simulink model "Wanderwellen_Leitungsmodell"  (R2022a)
settings: Solver=VariableStepAuto  StartTime=0.0  StopTime=0.05  RelTol=1e-3
model workspace (MAT data in the model file):
  C_impedanz = 1
  C_quelle = 1
  Delta_C = 2e-09
  Delta_G = 5000000
  Delta_L = 0.000228
  Delta_R = 0.048
  L_impedanz = 1
  L_quelle = 1
  R_impedanz = 0
  R_quelle = 0
  U = 20000
  U_type = 1
  Z_abschluss_type = 1
  Z_quelle_type = 1
  f = 50
  laenge = 0.2
  n_seg = 1
libraries: fl_lib x617, nesl_utility x207, ee_lib x3
(part 2 of 6)

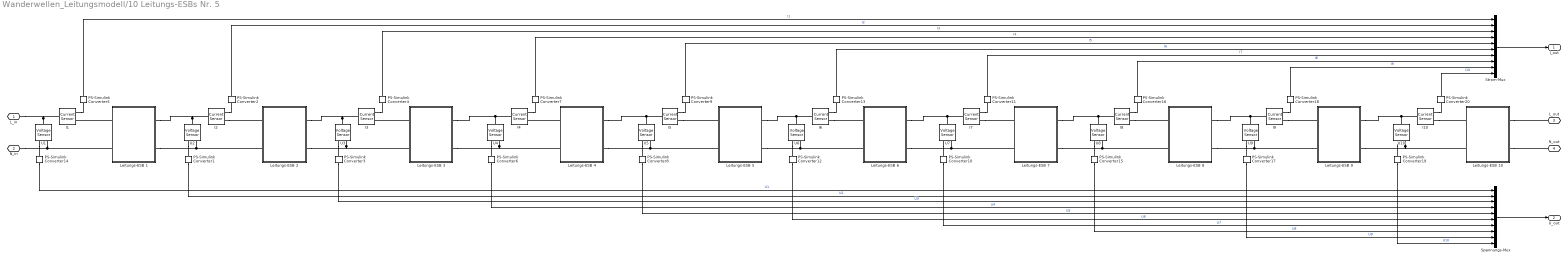
== system Wanderwellen_Leitungsmodell/10 Leitungs-ESBs Nr. 5 ==
  I{1..10} (10 alike) : fl_lib/Electrical/Electrical Sensors/Current Sensor
      settings: SourceProductBaseCode=PW,SS,VE
  Leitungs-ESB 1 : Subsystem
  Leitungs-ESB 10 : Subsystem
  Leitungs-ESB 2 : Subsystem
  Leitungs-ESB 3 : Subsystem
  Leitungs-ESB 4 : Subsystem
  Leitungs-ESB 5 : Subsystem
  Leitungs-ESB 6 : Subsystem
  Leitungs-ESB 7 : Subsystem
  Leitungs-ESB 8 : Subsystem
  Leitungs-ESB 9 : Subsystem
  PS-Simulink Converter{1..20} (20 alike) : nesl_utility/PS-Simulink Converter  PhysicalDomain=network_engine_domain  SubClassName=ps_output  LeftPortType=input  RightPortType=output  PseudoPeriodic=off  Frequencies=[]  VectorFormat=1-D array  Unit=inherit  AffineConversion=off
      settings: SourceProductBaseCode=SS,PW,VE
  Spannungs-Mux : Mux  Inputs=10
  Strom-Mux : Mux  Inputs=10
  U{1..10} (10 alike) : fl_lib/Electrical/Electrical Sensors/Voltage Sensor
      settings: SourceProductBaseCode=PW,SS,VE
  L_in : PMIOPort  Side=Left
  N_in : PMIOPort  Port=2  Side=Left
  L_out : PMIOPort  Port=3  Side=Right
  N_out : PMIOPort  Port=4  Side=Right
  I_out : Outport
  U_out : Outport  Port=2
  wires:
  PS-Simulink Converter5/1 -> Strom-Mux/1  "I1"
  PS-Simulink Converter2/1 -> Strom-Mux/2  "I2"
  PS-Simulink Converter4/1 -> Strom-Mux/3  "I3"
  PS-Simulink Converter7/1 -> Strom-Mux/4  "I4"
  PS-Simulink Converter9/1 -> Strom-Mux/5  "I5"
  PS-Simulink Converter13/1 -> Strom-Mux/6  "I6"
  PS-Simulink Converter11/1 -> Strom-Mux/7  "I7"
  PS-Simulink Converter16/1 -> Strom-Mux/8  "I8"
  PS-Simulink Converter18/1 -> Strom-Mux/9  "I9"
  PS-Simulink Converter20/1 -> Strom-Mux/10  "I10"
  PS-Simulink Converter19/1 -> Spannungs-Mux/10  "U10"
  PS-Simulink Converter17/1 -> Spannungs-Mux/9  "U9"
  PS-Simulink Converter15/1 -> Spannungs-Mux/8  "U8"
  PS-Simulink Converter10/1 -> Spannungs-Mux/7  "U7"
  PS-Simulink Converter12/1 -> Spannungs-Mux/6  "U6"
  PS-Simulink Converter8/1 -> Spannungs-Mux/5  "U5"
  PS-Simulink Converter6/1 -> Spannungs-Mux/4  "U4"
  PS-Simulink Converter3/1 -> Spannungs-Mux/3  "U3"
  PS-Simulink Converter1/1 -> Spannungs-Mux/2  "U2"
  PS-Simulink Converter14/1 -> Spannungs-Mux/1  "U1"
  Strom-Mux/1 -> I_out/1
  Spannungs-Mux/1 -> U_out/1
  connections:
  U1/LConn1 -- L_in/RConn1 -- I1/LConn1
  N_in/RConn1 -- Leitungs-ESB 1/LConn2 -- U1/RConn2
  Leitungs-ESB 1/LConn1 -- I1/RConn2
  I1/RConn1 -- PS-Simulink Converter5/LConn1
  U1/RConn1 -- PS-Simulink Converter14/LConn1
  Leitungs-ESB 2/LConn2 -- U2/RConn2 -- Leitungs-ESB 1/RConn2
  U2/LConn1 -- I2/LConn1 -- Leitungs-ESB 1/RConn1
  I2/RConn1 -- PS-Simulink Converter2/LConn1
  U2/RConn1 -- PS-Simulink Converter1/LConn1
  U3/RConn2 -- Leitungs-ESB 3/LConn2 -- Leitungs-ESB 2/RConn2
  U3/LConn1 -- I3/LConn1 -- Leitungs-ESB 2/RConn1
  I3/RConn1 -- PS-Simulink Converter4/LConn1
  U3/RConn1 -- PS-Simulink Converter3/LConn1
  Leitungs-ESB 3/LConn1 -- I3/RConn2
  U4/RConn2 -- Leitungs-ESB 3/RConn2 -- Leitungs-ESB 4/LConn2
  U4/LConn1 -- Leitungs-ESB 3/RConn1 -- I4/LConn1
  I4/RConn1 -- PS-Simulink Converter7/LConn1
  U4/RConn1 -- PS-Simulink Converter6/LConn1
  Leitungs-ESB 4/RConn2 -- Leitungs-ESB 5/LConn2 -- U5/RConn2
  Leitungs-ESB 4/RConn1 -- I5/LConn1 -- U5/LConn1
  I5/RConn1 -- PS-Simulink Converter9/LConn1
  U5/RConn1 -- PS-Simulink Converter8/LConn1
  Leitungs-ESB 6/RConn2 -- Leitungs-ESB 7/LConn2 -- U7/RConn2
  Leitungs-ESB 6/RConn1 -- I7/LConn1 -- U7/LConn1
  I7/RConn1 -- PS-Simulink Converter11/LConn1
  U7/RConn1 -- PS-Simulink Converter10/LConn1
  Leitungs-ESB 6/LConn2 -- Leitungs-ESB 5/RConn2 -- U6/RConn2
  Leitungs-ESB 5/RConn1 -- I6/LConn1 -- U6/LConn1
  U6/RConn1 -- PS-Simulink Converter12/LConn1
  I6/RConn1 -- PS-Simulink Converter13/LConn1
  I6/RConn2 -- Leitungs-ESB 6/LConn1
  Leitungs-ESB 8/LConn2 -- Leitungs-ESB 7/RConn2 -- U8/RConn2
  Leitungs-ESB 7/RConn1 -- I8/LConn1 -- U8/LConn1
  I8/RConn1 -- PS-Simulink Converter16/LConn1
  U8/RConn1 -- PS-Simulink Converter15/LConn1
  Leitungs-ESB 8/RConn2 -- Leitungs-ESB 9/LConn2 -- U9/RConn2
  Leitungs-ESB 8/RConn1 -- I9/LConn1 -- U9/LConn1
  I9/RConn1 -- PS-Simulink Converter18/LConn1
  U9/RConn1 -- PS-Simulink Converter17/LConn1
  U10/RConn2 -- Leitungs-ESB 9/RConn2 -- Leitungs-ESB 10/LConn2
  Leitungs-ESB 9/RConn1 -- I10/LConn1 -- U10/LConn1
  I10/RConn1 -- PS-Simulink Converter20/LConn1
  U10/RConn1 -- PS-Simulink Converter19/LConn1
  Leitungs-ESB 10/RConn1 -- L_out/RConn1
  Leitungs-ESB 10/RConn2 -- N_out/RConn1
  I2/RConn2 -- Leitungs-ESB 2/LConn1
  Leitungs-ESB 4/LConn1 -- I4/RConn2
  I5/RConn2 -- Leitungs-ESB 5/LConn1
  I7/RConn2 -- Leitungs-ESB 7/LConn1
  I8/RConn2 -- Leitungs-ESB 8/LConn1
  I9/RConn2 -- Leitungs-ESB 9/LConn1
  I10/RConn2 -- Leitungs-ESB 10/LConn1

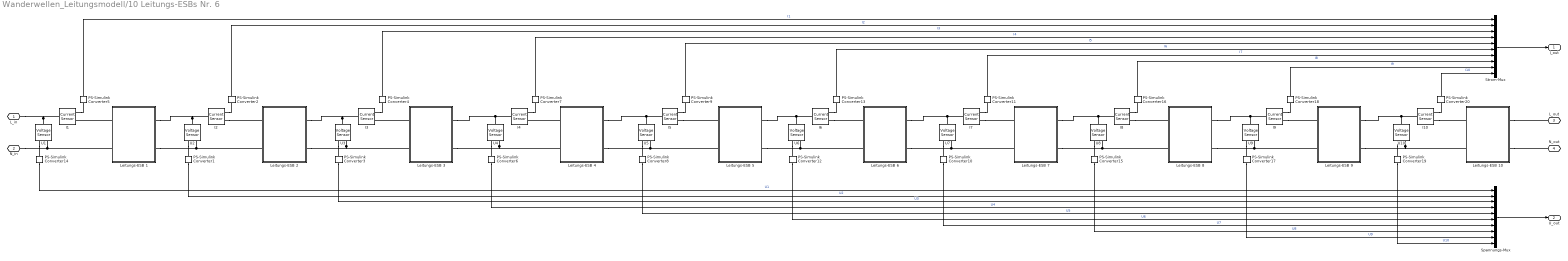
== system Wanderwellen_Leitungsmodell/10 Leitungs-ESBs Nr. 6 ==
  I{1..10} (10 alike) : fl_lib/Electrical/Electrical Sensors/Current Sensor
      settings: SourceProductBaseCode=PW,SS,VE
  Leitungs-ESB 1 : Subsystem
  Leitungs-ESB 10 : Subsystem
  Leitungs-ESB 2 : Subsystem
  Leitungs-ESB 3 : Subsystem
  Leitungs-ESB 4 : Subsystem
  Leitungs-ESB 5 : Subsystem
  Leitungs-ESB 6 : Subsystem
  Leitungs-ESB 7 : Subsystem
  Leitungs-ESB 8 : Subsystem
  Leitungs-ESB 9 : Subsystem
  PS-Simulink Converter{1..20} (20 alike) : nesl_utility/PS-Simulink Converter  PhysicalDomain=network_engine_domain  SubClassName=ps_output  LeftPortType=input  RightPortType=output  PseudoPeriodic=off  Frequencies=[]  VectorFormat=1-D array  Unit=inherit  AffineConversion=off
      settings: SourceProductBaseCode=SS,PW,VE
  Spannungs-Mux : Mux  Inputs=10
  Strom-Mux : Mux  Inputs=10
  U{1..10} (10 alike) : fl_lib/Electrical/Electrical Sensors/Voltage Sensor
      settings: SourceProductBaseCode=PW,SS,VE
  L_in : PMIOPort  Side=Left
  N_in : PMIOPort  Port=2  Side=Left
  L_out : PMIOPort  Port=3  Side=Right
  N_out : PMIOPort  Port=4  Side=Right
  I_out : Outport
  U_out : Outport  Port=2
  wires:
  PS-Simulink Converter5/1 -> Strom-Mux/1  "I1"
  PS-Simulink Converter2/1 -> Strom-Mux/2  "I2"
  PS-Simulink Converter4/1 -> Strom-Mux/3  "I3"
  PS-Simulink Converter7/1 -> Strom-Mux/4  "I4"
  PS-Simulink Converter9/1 -> Strom-Mux/5  "I5"
  PS-Simulink Converter13/1 -> Strom-Mux/6  "I6"
  PS-Simulink Converter11/1 -> Strom-Mux/7  "I7"
  PS-Simulink Converter16/1 -> Strom-Mux/8  "I8"
  PS-Simulink Converter18/1 -> Strom-Mux/9  "I9"
  PS-Simulink Converter20/1 -> Strom-Mux/10  "I10"
  PS-Simulink Converter19/1 -> Spannungs-Mux/10  "U10"
  PS-Simulink Converter17/1 -> Spannungs-Mux/9  "U9"
  PS-Simulink Converter15/1 -> Spannungs-Mux/8  "U8"
  PS-Simulink Converter10/1 -> Spannungs-Mux/7  "U7"
  PS-Simulink Converter12/1 -> Spannungs-Mux/6  "U6"
  PS-Simulink Converter8/1 -> Spannungs-Mux/5  "U5"
  PS-Simulink Converter6/1 -> Spannungs-Mux/4  "U4"
  PS-Simulink Converter3/1 -> Spannungs-Mux/3  "U3"
  PS-Simulink Converter1/1 -> Spannungs-Mux/2  "U2"
  PS-Simulink Converter14/1 -> Spannungs-Mux/1  "U1"
  Strom-Mux/1 -> I_out/1
  Spannungs-Mux/1 -> U_out/1
  connections:
  U1/LConn1 -- L_in/RConn1 -- I1/LConn1
  N_in/RConn1 -- Leitungs-ESB 1/LConn2 -- U1/RConn2
  Leitungs-ESB 1/LConn1 -- I1/RConn2
  I1/RConn1 -- PS-Simulink Converter5/LConn1
  U1/RConn1 -- PS-Simulink Converter14/LConn1
  Leitungs-ESB 2/LConn2 -- U2/RConn2 -- Leitungs-ESB 1/RConn2
  U2/LConn1 -- I2/LConn1 -- Leitungs-ESB 1/RConn1
  I2/RConn1 -- PS-Simulink Converter2/LConn1
  U2/RConn1 -- PS-Simulink Converter1/LConn1
  U3/RConn2 -- Leitungs-ESB 3/LConn2 -- Leitungs-ESB 2/RConn2
  U3/LConn1 -- I3/LConn1 -- Leitungs-ESB 2/RConn1
  I3/RConn1 -- PS-Simulink Converter4/LConn1
  U3/RConn1 -- PS-Simulink Converter3/LConn1
  Leitungs-ESB 3/LConn1 -- I3/RConn2
  U4/RConn2 -- Leitungs-ESB 3/RConn2 -- Leitungs-ESB 4/LConn2
  U4/LConn1 -- Leitungs-ESB 3/RConn1 -- I4/LConn1
  I4/RConn1 -- PS-Simulink Converter7/LConn1
  U4/RConn1 -- PS-Simulink Converter6/LConn1
  Leitungs-ESB 4/RConn2 -- Leitungs-ESB 5/LConn2 -- U5/RConn2
  Leitungs-ESB 4/RConn1 -- I5/LConn1 -- U5/LConn1
  I5/RConn1 -- PS-Simulink Converter9/LConn1
  U5/RConn1 -- PS-Simulink Converter8/LConn1
  Leitungs-ESB 6/RConn2 -- Leitungs-ESB 7/LConn2 -- U7/RConn2
  Leitungs-ESB 6/RConn1 -- I7/LConn1 -- U7/LConn1
  I7/RConn1 -- PS-Simulink Converter11/LConn1
  U7/RConn1 -- PS-Simulink Converter10/LConn1
  Leitungs-ESB 6/LConn2 -- Leitungs-ESB 5/RConn2 -- U6/RConn2
  Leitungs-ESB 5/RConn1 -- I6/LConn1 -- U6/LConn1
  U6/RConn1 -- PS-Simulink Converter12/LConn1
  I6/RConn1 -- PS-Simulink Converter13/LConn1
  I6/RConn2 -- Leitungs-ESB 6/LConn1
  Leitungs-ESB 8/LConn2 -- Leitungs-ESB 7/RConn2 -- U8/RConn2
  Leitungs-ESB 7/RConn1 -- I8/LConn1 -- U8/LConn1
  I8/RConn1 -- PS-Simulink Converter16/LConn1
  U8/RConn1 -- PS-Simulink Converter15/LConn1
  Leitungs-ESB 8/RConn2 -- Leitungs-ESB 9/LConn2 -- U9/RConn2
  Leitungs-ESB 8/RConn1 -- I9/LConn1 -- U9/LConn1
  I9/RConn1 -- PS-Simulink Converter18/LConn1
  U9/RConn1 -- PS-Simulink Converter17/LConn1
  U10/RConn2 -- Leitungs-ESB 9/RConn2 -- Leitungs-ESB 10/LConn2
  Leitungs-ESB 9/RConn1 -- I10/LConn1 -- U10/LConn1
  I10/RConn1 -- PS-Simulink Converter20/LConn1
  U10/RConn1 -- PS-Simulink Converter19/LConn1
  Leitungs-ESB 10/RConn1 -- L_out/RConn1
  Leitungs-ESB 10/RConn2 -- N_out/RConn1
  I2/RConn2 -- Leitungs-ESB 2/LConn1
  Leitungs-ESB 4/LConn1 -- I4/RConn2
  I5/RConn2 -- Leitungs-ESB 5/LConn1
  I7/RConn2 -- Leitungs-ESB 7/LConn1
  I8/RConn2 -- Leitungs-ESB 8/LConn1
  I9/RConn2 -- Leitungs-ESB 9/LConn1
  I10/RConn2 -- Leitungs-ESB 10/LConn1

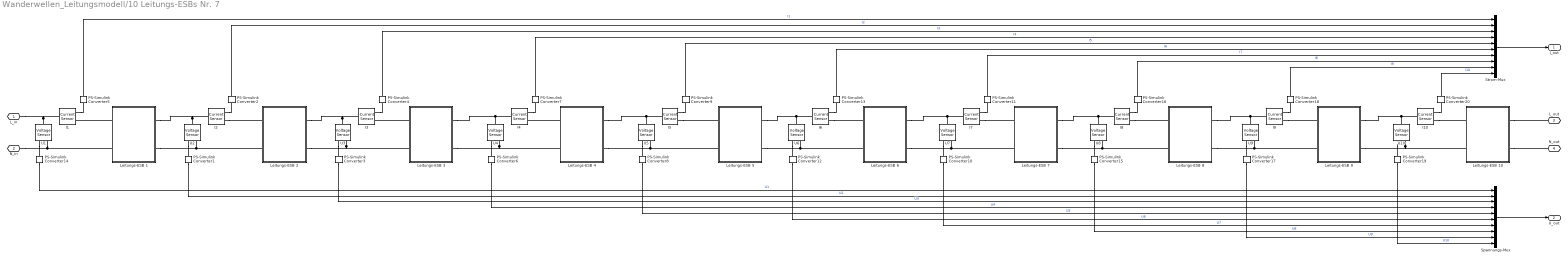
== system Wanderwellen_Leitungsmodell/10 Leitungs-ESBs Nr. 7 ==
  I{1..10} (10 alike) : fl_lib/Electrical/Electrical Sensors/Current Sensor
      settings: SourceProductBaseCode=PW,SS,VE
  Leitungs-ESB 1 : Subsystem
  Leitungs-ESB 10 : Subsystem
  Leitungs-ESB 2 : Subsystem
  Leitungs-ESB 3 : Subsystem
  Leitungs-ESB 4 : Subsystem
  Leitungs-ESB 5 : Subsystem
  Leitungs-ESB 6 : Subsystem
  Leitungs-ESB 7 : Subsystem
  Leitungs-ESB 8 : Subsystem
  Leitungs-ESB 9 : Subsystem
  PS-Simulink Converter{1..20} (20 alike) : nesl_utility/PS-Simulink Converter  PhysicalDomain=network_engine_domain  SubClassName=ps_output  LeftPortType=input  RightPortType=output  PseudoPeriodic=off  Frequencies=[]  VectorFormat=1-D array  Unit=inherit  AffineConversion=off
      settings: SourceProductBaseCode=SS,PW,VE
  Spannungs-Mux : Mux  Inputs=10
  Strom-Mux : Mux  Inputs=10
  U{1..10} (10 alike) : fl_lib/Electrical/Electrical Sensors/Voltage Sensor
      settings: SourceProductBaseCode=PW,SS,VE
  L_in : PMIOPort  Side=Left
  N_in : PMIOPort  Port=2  Side=Left
  L_out : PMIOPort  Port=3  Side=Right
  N_out : PMIOPort  Port=4  Side=Right
  I_out : Outport
  U_out : Outport  Port=2
  wires:
  PS-Simulink Converter5/1 -> Strom-Mux/1  "I1"
  PS-Simulink Converter2/1 -> Strom-Mux/2  "I2"
  PS-Simulink Converter4/1 -> Strom-Mux/3  "I3"
  PS-Simulink Converter7/1 -> Strom-Mux/4  "I4"
  PS-Simulink Converter9/1 -> Strom-Mux/5  "I5"
  PS-Simulink Converter13/1 -> Strom-Mux/6  "I6"
  PS-Simulink Converter11/1 -> Strom-Mux/7  "I7"
  PS-Simulink Converter16/1 -> Strom-Mux/8  "I8"
  PS-Simulink Converter18/1 -> Strom-Mux/9  "I9"
  PS-Simulink Converter20/1 -> Strom-Mux/10  "I10"
  PS-Simulink Converter19/1 -> Spannungs-Mux/10  "U10"
  PS-Simulink Converter17/1 -> Spannungs-Mux/9  "U9"
  PS-Simulink Converter15/1 -> Spannungs-Mux/8  "U8"
  PS-Simulink Converter10/1 -> Spannungs-Mux/7  "U7"
  PS-Simulink Converter12/1 -> Spannungs-Mux/6  "U6"
  PS-Simulink Converter8/1 -> Spannungs-Mux/5  "U5"
  PS-Simulink Converter6/1 -> Spannungs-Mux/4  "U4"
  PS-Simulink Converter3/1 -> Spannungs-Mux/3  "U3"
  PS-Simulink Converter1/1 -> Spannungs-Mux/2  "U2"
  PS-Simulink Converter14/1 -> Spannungs-Mux/1  "U1"
  Strom-Mux/1 -> I_out/1
  Spannungs-Mux/1 -> U_out/1
  connections:
  U1/LConn1 -- L_in/RConn1 -- I1/LConn1
  N_in/RConn1 -- Leitungs-ESB 1/LConn2 -- U1/RConn2
  Leitungs-ESB 1/LConn1 -- I1/RConn2
  I1/RConn1 -- PS-Simulink Converter5/LConn1
  U1/RConn1 -- PS-Simulink Converter14/LConn1
  Leitungs-ESB 2/LConn2 -- U2/RConn2 -- Leitungs-ESB 1/RConn2
  U2/LConn1 -- I2/LConn1 -- Leitungs-ESB 1/RConn1
  I2/RConn1 -- PS-Simulink Converter2/LConn1
  U2/RConn1 -- PS-Simulink Converter1/LConn1
  U3/RConn2 -- Leitungs-ESB 3/LConn2 -- Leitungs-ESB 2/RConn2
  U3/LConn1 -- I3/LConn1 -- Leitungs-ESB 2/RConn1
  I3/RConn1 -- PS-Simulink Converter4/LConn1
  U3/RConn1 -- PS-Simulink Converter3/LConn1
  Leitungs-ESB 3/LConn1 -- I3/RConn2
  U4/RConn2 -- Leitungs-ESB 3/RConn2 -- Leitungs-ESB 4/LConn2
  U4/LConn1 -- Leitungs-ESB 3/RConn1 -- I4/LConn1
  I4/RConn1 -- PS-Simulink Converter7/LConn1
  U4/RConn1 -- PS-Simulink Converter6/LConn1
  Leitungs-ESB 4/RConn2 -- Leitungs-ESB 5/LConn2 -- U5/RConn2
  Leitungs-ESB 4/RConn1 -- I5/LConn1 -- U5/LConn1
  I5/RConn1 -- PS-Simulink Converter9/LConn1
  U5/RConn1 -- PS-Simulink Converter8/LConn1
  Leitungs-ESB 6/RConn2 -- Leitungs-ESB 7/LConn2 -- U7/RConn2
  Leitungs-ESB 6/RConn1 -- I7/LConn1 -- U7/LConn1
  I7/RConn1 -- PS-Simulink Converter11/LConn1
  U7/RConn1 -- PS-Simulink Converter10/LConn1
  Leitungs-ESB 6/LConn2 -- Leitungs-ESB 5/RConn2 -- U6/RConn2
  Leitungs-ESB 5/RConn1 -- I6/LConn1 -- U6/LConn1
  U6/RConn1 -- PS-Simulink Converter12/LConn1
  I6/RConn1 -- PS-Simulink Converter13/LConn1
  I6/RConn2 -- Leitungs-ESB 6/LConn1
  Leitungs-ESB 8/LConn2 -- Leitungs-ESB 7/RConn2 -- U8/RConn2
  Leitungs-ESB 7/RConn1 -- I8/LConn1 -- U8/LConn1
  I8/RConn1 -- PS-Simulink Converter16/LConn1
  U8/RConn1 -- PS-Simulink Converter15/LConn1
  Leitungs-ESB 8/RConn2 -- Leitungs-ESB 9/LConn2 -- U9/RConn2
  Leitungs-ESB 8/RConn1 -- I9/LConn1 -- U9/LConn1
  I9/RConn1 -- PS-Simulink Converter18/LConn1
  U9/RConn1 -- PS-Simulink Converter17/LConn1
  U10/RConn2 -- Leitungs-ESB 9/RConn2 -- Leitungs-ESB 10/LConn2
  Leitungs-ESB 9/RConn1 -- I10/LConn1 -- U10/LConn1
  I10/RConn1 -- PS-Simulink Converter20/LConn1
  U10/RConn1 -- PS-Simulink Converter19/LConn1
  Leitungs-ESB 10/RConn1 -- L_out/RConn1
  Leitungs-ESB 10/RConn2 -- N_out/RConn1
  I2/RConn2 -- Leitungs-ESB 2/LConn1
  Leitungs-ESB 4/LConn1 -- I4/RConn2
  I5/RConn2 -- Leitungs-ESB 5/LConn1
  I7/RConn2 -- Leitungs-ESB 7/LConn1
  I8/RConn2 -- Leitungs-ESB 8/LConn1
  I9/RConn2 -- Leitungs-ESB 9/LConn1
  I10/RConn2 -- Leitungs-ESB 10/LConn1

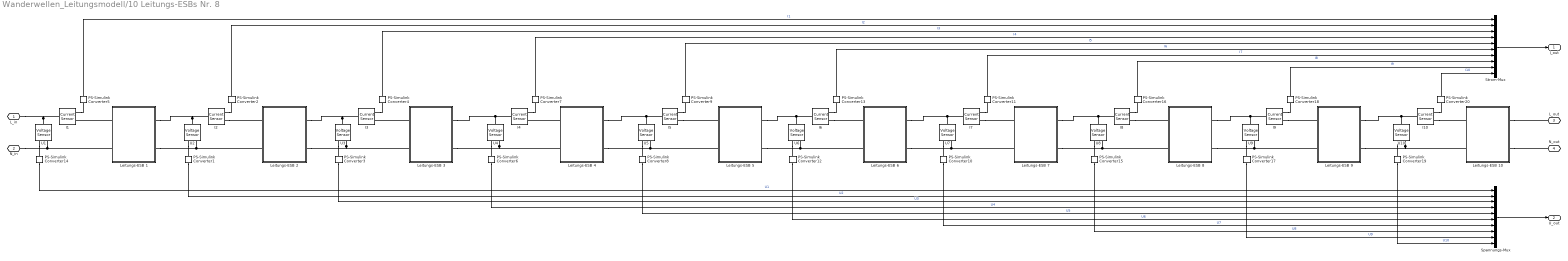
== system Wanderwellen_Leitungsmodell/10 Leitungs-ESBs Nr. 8 ==
  I{1..10} (10 alike) : fl_lib/Electrical/Electrical Sensors/Current Sensor
      settings: SourceProductBaseCode=PW,SS,VE
  Leitungs-ESB 1 : Subsystem
  Leitungs-ESB 10 : Subsystem
  Leitungs-ESB 2 : Subsystem
  Leitungs-ESB 3 : Subsystem
  Leitungs-ESB 4 : Subsystem
  Leitungs-ESB 5 : Subsystem
  Leitungs-ESB 6 : Subsystem
  Leitungs-ESB 7 : Subsystem
  Leitungs-ESB 8 : Subsystem
  Leitungs-ESB 9 : Subsystem
  PS-Simulink Converter{1..20} (20 alike) : nesl_utility/PS-Simulink Converter  PhysicalDomain=network_engine_domain  SubClassName=ps_output  LeftPortType=input  RightPortType=output  PseudoPeriodic=off  Frequencies=[]  VectorFormat=1-D array  Unit=inherit  AffineConversion=off
      settings: SourceProductBaseCode=SS,PW,VE
  Spannungs-Mux : Mux  Inputs=10
  Strom-Mux : Mux  Inputs=10
  U{1..10} (10 alike) : fl_lib/Electrical/Electrical Sensors/Voltage Sensor
      settings: SourceProductBaseCode=PW,SS,VE
  L_in : PMIOPort  Side=Left
  N_in : PMIOPort  Port=2  Side=Left
  L_out : PMIOPort  Port=3  Side=Right
  N_out : PMIOPort  Port=4  Side=Right
  I_out : Outport
  U_out : Outport  Port=2
  wires:
  PS-Simulink Converter5/1 -> Strom-Mux/1  "I1"
  PS-Simulink Converter2/1 -> Strom-Mux/2  "I2"
  PS-Simulink Converter4/1 -> Strom-Mux/3  "I3"
  PS-Simulink Converter7/1 -> Strom-Mux/4  "I4"
  PS-Simulink Converter9/1 -> Strom-Mux/5  "I5"
  PS-Simulink Converter13/1 -> Strom-Mux/6  "I6"
  PS-Simulink Converter11/1 -> Strom-Mux/7  "I7"
  PS-Simulink Converter16/1 -> Strom-Mux/8  "I8"
  PS-Simulink Converter18/1 -> Strom-Mux/9  "I9"
  PS-Simulink Converter20/1 -> Strom-Mux/10  "I10"
  PS-Simulink Converter19/1 -> Spannungs-Mux/10  "U10"
  PS-Simulink Converter17/1 -> Spannungs-Mux/9  "U9"
  PS-Simulink Converter15/1 -> Spannungs-Mux/8  "U8"
  PS-Simulink Converter10/1 -> Spannungs-Mux/7  "U7"
  PS-Simulink Converter12/1 -> Spannungs-Mux/6  "U6"
  PS-Simulink Converter8/1 -> Spannungs-Mux/5  "U5"
  PS-Simulink Converter6/1 -> Spannungs-Mux/4  "U4"
  PS-Simulink Converter3/1 -> Spannungs-Mux/3  "U3"
  PS-Simulink Converter1/1 -> Spannungs-Mux/2  "U2"
  PS-Simulink Converter14/1 -> Spannungs-Mux/1  "U1"
  Strom-Mux/1 -> I_out/1
  Spannungs-Mux/1 -> U_out/1
  connections:
  U1/LConn1 -- L_in/RConn1 -- I1/LConn1
  N_in/RConn1 -- Leitungs-ESB 1/LConn2 -- U1/RConn2
  Leitungs-ESB 1/LConn1 -- I1/RConn2
  I1/RConn1 -- PS-Simulink Converter5/LConn1
  U1/RConn1 -- PS-Simulink Converter14/LConn1
  Leitungs-ESB 2/LConn2 -- U2/RConn2 -- Leitungs-ESB 1/RConn2
  U2/LConn1 -- I2/LConn1 -- Leitungs-ESB 1/RConn1
  I2/RConn1 -- PS-Simulink Converter2/LConn1
  U2/RConn1 -- PS-Simulink Converter1/LConn1
  U3/RConn2 -- Leitungs-ESB 3/LConn2 -- Leitungs-ESB 2/RConn2
  U3/LConn1 -- I3/LConn1 -- Leitungs-ESB 2/RConn1
  I3/RConn1 -- PS-Simulink Converter4/LConn1
  U3/RConn1 -- PS-Simulink Converter3/LConn1
  Leitungs-ESB 3/LConn1 -- I3/RConn2
  U4/RConn2 -- Leitungs-ESB 3/RConn2 -- Leitungs-ESB 4/LConn2
  U4/LConn1 -- Leitungs-ESB 3/RConn1 -- I4/LConn1
  I4/RConn1 -- PS-Simulink Converter7/LConn1
  U4/RConn1 -- PS-Simulink Converter6/LConn1
  Leitungs-ESB 4/RConn2 -- Leitungs-ESB 5/LConn2 -- U5/RConn2
  Leitungs-ESB 4/RConn1 -- I5/LConn1 -- U5/LConn1
  I5/RConn1 -- PS-Simulink Converter9/LConn1
  U5/RConn1 -- PS-Simulink Converter8/LConn1
  Leitungs-ESB 6/RConn2 -- Leitungs-ESB 7/LConn2 -- U7/RConn2
  Leitungs-ESB 6/RConn1 -- I7/LConn1 -- U7/LConn1
  I7/RConn1 -- PS-Simulink Converter11/LConn1
  U7/RConn1 -- PS-Simulink Converter10/LConn1
  Leitungs-ESB 6/LConn2 -- Leitungs-ESB 5/RConn2 -- U6/RConn2
  Leitungs-ESB 5/RConn1 -- I6/LConn1 -- U6/LConn1
  U6/RConn1 -- PS-Simulink Converter12/LConn1
  I6/RConn1 -- PS-Simulink Converter13/LConn1
  I6/RConn2 -- Leitungs-ESB 6/LConn1
  Leitungs-ESB 8/LConn2 -- Leitungs-ESB 7/RConn2 -- U8/RConn2
  Leitungs-ESB 7/RConn1 -- I8/LConn1 -- U8/LConn1
  I8/RConn1 -- PS-Simulink Converter16/LConn1
  U8/RConn1 -- PS-Simulink Converter15/LConn1
  Leitungs-ESB 8/RConn2 -- Leitungs-ESB 9/LConn2 -- U9/RConn2
  Leitungs-ESB 8/RConn1 -- I9/LConn1 -- U9/LConn1
  I9/RConn1 -- PS-Simulink Converter18/LConn1
  U9/RConn1 -- PS-Simulink Converter17/LConn1
  U10/RConn2 -- Leitungs-ESB 9/RConn2 -- Leitungs-ESB 10/LConn2
  Leitungs-ESB 9/RConn1 -- I10/LConn1 -- U10/LConn1
  I10/RConn1 -- PS-Simulink Converter20/LConn1
  U10/RConn1 -- PS-Simulink Converter19/LConn1
  Leitungs-ESB 10/RConn1 -- L_out/RConn1
  Leitungs-ESB 10/RConn2 -- N_out/RConn1
  I2/RConn2 -- Leitungs-ESB 2/LConn1
  Leitungs-ESB 4/LConn1 -- I4/RConn2
  I5/RConn2 -- Leitungs-ESB 5/LConn1
  I7/RConn2 -- Leitungs-ESB 7/LConn1
  I8/RConn2 -- Leitungs-ESB 8/LConn1
  I9/RConn2 -- Leitungs-ESB 9/LConn1
  I10/RConn2 -- Leitungs-ESB 10/LConn1

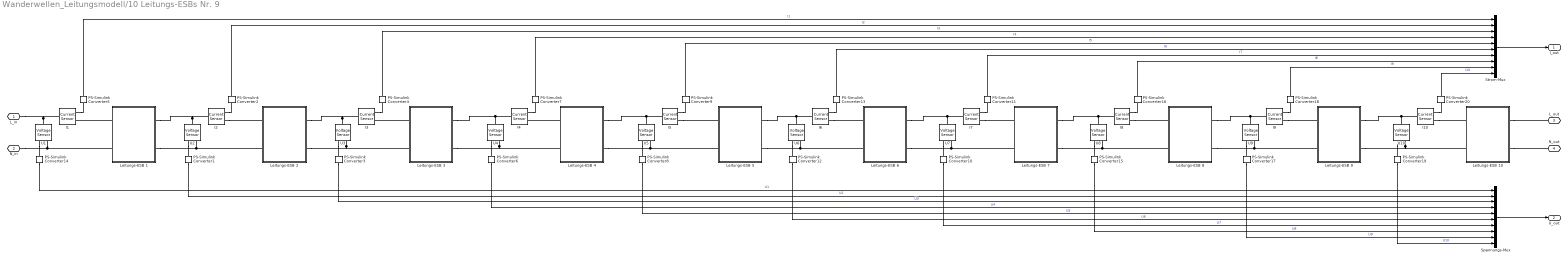
== system Wanderwellen_Leitungsmodell/10 Leitungs-ESBs Nr. 9 ==
  I{1..10} (10 alike) : fl_lib/Electrical/Electrical Sensors/Current Sensor
      settings: SourceProductBaseCode=PW,SS,VE
  Leitungs-ESB 1 : Subsystem
  Leitungs-ESB 10 : Subsystem
  Leitungs-ESB 2 : Subsystem
  Leitungs-ESB 3 : Subsystem
  Leitungs-ESB 4 : Subsystem
  Leitungs-ESB 5 : Subsystem
  Leitungs-ESB 6 : Subsystem
  Leitungs-ESB 7 : Subsystem
  Leitungs-ESB 8 : Subsystem
  Leitungs-ESB 9 : Subsystem
  PS-Simulink Converter{1..20} (20 alike) : nesl_utility/PS-Simulink Converter  PhysicalDomain=network_engine_domain  SubClassName=ps_output  LeftPortType=input  RightPortType=output  PseudoPeriodic=off  Frequencies=[]  VectorFormat=1-D array  Unit=inherit  AffineConversion=off
      settings: SourceProductBaseCode=SS,PW,VE
  Spannungs-Mux : Mux  Inputs=10
  Strom-Mux : Mux  Inputs=10
  U{1..10} (10 alike) : fl_lib/Electrical/Electrical Sensors/Voltage Sensor
      settings: SourceProductBaseCode=PW,SS,VE
  L_in : PMIOPort  Side=Left
  N_in : PMIOPort  Port=2  Side=Left
  L_out : PMIOPort  Port=3  Side=Right
  N_out : PMIOPort  Port=4  Side=Right
  I_out : Outport
  U_out : Outport  Port=2
  wires:
  PS-Simulink Converter5/1 -> Strom-Mux/1  "I1"
  PS-Simulink Converter2/1 -> Strom-Mux/2  "I2"
  PS-Simulink Converter4/1 -> Strom-Mux/3  "I3"
  PS-Simulink Converter7/1 -> Strom-Mux/4  "I4"
  PS-Simulink Converter9/1 -> Strom-Mux/5  "I5"
  PS-Simulink Converter13/1 -> Strom-Mux/6  "I6"
  PS-Simulink Converter11/1 -> Strom-Mux/7  "I7"
  PS-Simulink Converter16/1 -> Strom-Mux/8  "I8"
  PS-Simulink Converter18/1 -> Strom-Mux/9  "I9"
  PS-Simulink Converter20/1 -> Strom-Mux/10  "I10"
  PS-Simulink Converter19/1 -> Spannungs-Mux/10  "U10"
  PS-Simulink Converter17/1 -> Spannungs-Mux/9  "U9"
  PS-Simulink Converter15/1 -> Spannungs-Mux/8  "U8"
  PS-Simulink Converter10/1 -> Spannungs-Mux/7  "U7"
  PS-Simulink Converter12/1 -> Spannungs-Mux/6  "U6"
  PS-Simulink Converter8/1 -> Spannungs-Mux/5  "U5"
  PS-Simulink Converter6/1 -> Spannungs-Mux/4  "U4"
  PS-Simulink Converter3/1 -> Spannungs-Mux/3  "U3"
  PS-Simulink Converter1/1 -> Spannungs-Mux/2  "U2"
  PS-Simulink Converter14/1 -> Spannungs-Mux/1  "U1"
  Strom-Mux/1 -> I_out/1
  Spannungs-Mux/1 -> U_out/1
  connections:
  U1/LConn1 -- L_in/RConn1 -- I1/LConn1
  N_in/RConn1 -- Leitungs-ESB 1/LConn2 -- U1/RConn2
  Leitungs-ESB 1/LConn1 -- I1/RConn2
  I1/RConn1 -- PS-Simulink Converter5/LConn1
  U1/RConn1 -- PS-Simulink Converter14/LConn1
  Leitungs-ESB 2/LConn2 -- U2/RConn2 -- Leitungs-ESB 1/RConn2
  U2/LConn1 -- I2/LConn1 -- Leitungs-ESB 1/RConn1
  I2/RConn1 -- PS-Simulink Converter2/LConn1
  U2/RConn1 -- PS-Simulink Converter1/LConn1
  U3/RConn2 -- Leitungs-ESB 3/LConn2 -- Leitungs-ESB 2/RConn2
  U3/LConn1 -- I3/LConn1 -- Leitungs-ESB 2/RConn1
  I3/RConn1 -- PS-Simulink Converter4/LConn1
  U3/RConn1 -- PS-Simulink Converter3/LConn1
  Leitungs-ESB 3/LConn1 -- I3/RConn2
  U4/RConn2 -- Leitungs-ESB 3/RConn2 -- Leitungs-ESB 4/LConn2
  U4/LConn1 -- Leitungs-ESB 3/RConn1 -- I4/LConn1
  I4/RConn1 -- PS-Simulink Converter7/LConn1
  U4/RConn1 -- PS-Simulink Converter6/LConn1
  Leitungs-ESB 4/RConn2 -- Leitungs-ESB 5/LConn2 -- U5/RConn2
  Leitungs-ESB 4/RConn1 -- I5/LConn1 -- U5/LConn1
  I5/RConn1 -- PS-Simulink Converter9/LConn1
  U5/RConn1 -- PS-Simulink Converter8/LConn1
  Leitungs-ESB 6/RConn2 -- Leitungs-ESB 7/LConn2 -- U7/RConn2
  Leitungs-ESB 6/RConn1 -- I7/LConn1 -- U7/LConn1
  I7/RConn1 -- PS-Simulink Converter11/LConn1
  U7/RConn1 -- PS-Simulink Converter10/LConn1
  Leitungs-ESB 6/LConn2 -- Leitungs-ESB 5/RConn2 -- U6/RConn2
  Leitungs-ESB 5/RConn1 -- I6/LConn1 -- U6/LConn1
  U6/RConn1 -- PS-Simulink Converter12/LConn1
  I6/RConn1 -- PS-Simulink Converter13/LConn1
  I6/RConn2 -- Leitungs-ESB 6/LConn1
  Leitungs-ESB 8/LConn2 -- Leitungs-ESB 7/RConn2 -- U8/RConn2
  Leitungs-ESB 7/RConn1 -- I8/LConn1 -- U8/LConn1
  I8/RConn1 -- PS-Simulink Converter16/LConn1
  U8/RConn1 -- PS-Simulink Converter15/LConn1
  Leitungs-ESB 8/RConn2 -- Leitungs-ESB 9/LConn2 -- U9/RConn2
  Leitungs-ESB 8/RConn1 -- I9/LConn1 -- U9/LConn1
  I9/RConn1 -- PS-Simulink Converter18/LConn1
  U9/RConn1 -- PS-Simulink Converter17/LConn1
  U10/RConn2 -- Leitungs-ESB 9/RConn2 -- Leitungs-ESB 10/LConn2
  Leitungs-ESB 9/RConn1 -- I10/LConn1 -- U10/LConn1
  I10/RConn1 -- PS-Simulink Converter20/LConn1
  U10/RConn1 -- PS-Simulink Converter19/LConn1
  Leitungs-ESB 10/RConn1 -- L_out/RConn1
  Leitungs-ESB 10/RConn2 -- N_out/RConn1
  I2/RConn2 -- Leitungs-ESB 2/LConn1
  Leitungs-ESB 4/LConn1 -- I4/RConn2
  I5/RConn2 -- Leitungs-ESB 5/LConn1
  I7/RConn2 -- Leitungs-ESB 7/LConn1
  I8/RConn2 -- Leitungs-ESB 8/LConn1
  I9/RConn2 -- Leitungs-ESB 9/LConn1
  I10/RConn2 -- Leitungs-ESB 10/LConn1

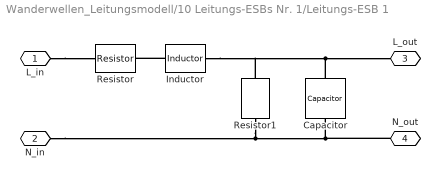
== system Wanderwellen_Leitungsmodell/10 Leitungs-ESBs Nr. 1/Leitungs-ESB 1 ==
  Capacitor : fl_lib/Electrical/Electrical Elements/Capacitor  c=Delta_C F  r=1e-6 Ohm  g=0 1/Ohm  i_specify=off  i_priority=None  i=0 A  i_nominal_specify=off  i_nominal_unit=A  i_nominal_value=1  v_specify=off  v_priority=None  v=0 V  v_nominal_specify=off  v_nominal_unit=V  v_nominal_value=1  vc_specify=off  vc_priority=High  vc=0 V  vc_nominal_specify=off  vc_nominal_unit=V  vc_nominal_value=1
      settings: SourceProductBaseCode=PW,SS,VE
  Inductor : fl_lib/Electrical/Electrical Elements/Inductor  l=Delta_L H  r=0 Ohm  g=1e-9 1/Ohm  i_specify=off  i_priority=None  i=0 A  i_nominal_specify=off  i_nominal_unit=A  i_nominal_value=1  v_specify=off  v_priority=None  v=0 V  v_nominal_specify=off  v_nominal_unit=V  v_nominal_value=1  i_L_specify=off  i_L_priority=High  i_L=0 A  i_L_nominal_specify=off  i_L_nominal_unit=A  i_L_nominal_value=1
      settings: SourceProductBaseCode=PW,SS,VE
  Resistor : fl_lib/Electrical/Electrical Elements/Resistor  R=Delta_R Ohm  i_specify=off  i_priority=None  i=0 A  i_nominal_specify=off  i_nominal_unit=A  i_nominal_value=1  v_specify=off  v_priority=None  v=0 V  v_nominal_specify=off  v_nominal_unit=V  v_nominal_value=1
      settings: SourceProductBaseCode=PW,SS,VE
  Resistor1 : fl_lib/Electrical/Electrical Elements/Resistor  R=Delta_G Ohm  i_specify=off  i_priority=None  i=0 A  i_nominal_specify=off  i_nominal_unit=A  i_nominal_value=1  v_specify=off  v_priority=None  v=0 V  v_nominal_specify=off  v_nominal_unit=V  v_nominal_value=1
      settings: SourceProductBaseCode=PW,SS,VE
  L_in : PMIOPort  Side=Left
  N_in : PMIOPort  Port=2  Side=Left
  L_out : PMIOPort  Port=3  Side=Right
  N_out : PMIOPort  Port=4  Side=Right
  connections:
  Capacitor/LConn1 -- Resistor1/LConn1 -- Inductor/RConn1 -- L_out/RConn1
  Inductor/LConn1 -- Resistor/RConn1
  L_in/RConn1 -- Resistor/LConn1
  Resistor1/RConn1 -- N_in/RConn1 -- N_out/RConn1 -- Capacitor/RConn1

== system Wanderwellen_Leitungsmodell/10 Leitungs-ESBs Nr. 1/Leitungs-ESB 10 ==
  Capacitor : fl_lib/Electrical/Electrical Elements/Capacitor  c=Delta_C F  r=1e-6 Ohm  g=0 1/Ohm  i_specify=off  i_priority=None  i=0 A  i_nominal_specify=off  i_nominal_unit=A  i_nominal_value=1  v_specify=off  v_priority=None  v=0 V  v_nominal_specify=off  v_nominal_unit=V  v_nominal_value=1  vc_specify=off  vc_priority=High  vc=0 V  vc_nominal_specify=off  vc_nominal_unit=V  vc_nominal_value=1
      settings: SourceProductBaseCode=PW,SS,VE
  Inductor : fl_lib/Electrical/Electrical Elements/Inductor  l=Delta_L H  r=0 Ohm  g=1e-9 1/Ohm  i_specify=off  i_priority=None  i=0 A  i_nominal_specify=off  i_nominal_unit=A  i_nominal_value=1  v_specify=off  v_priority=None  v=0 V  v_nominal_specify=off  v_nominal_unit=V  v_nominal_value=1  i_L_specify=off  i_L_priority=High  i_L=0 A  i_L_nominal_specify=off  i_L_nominal_unit=A  i_L_nominal_value=1
      settings: SourceProductBaseCode=PW,SS,VE
  Resistor : fl_lib/Electrical/Electrical Elements/Resistor  R=Delta_R Ohm  i_specify=off  i_priority=None  i=0 A  i_nominal_specify=off  i_nominal_unit=A  i_nominal_value=1  v_specify=off  v_priority=None  v=0 V  v_nominal_specify=off  v_nominal_unit=V  v_nominal_value=1
      settings: SourceProductBaseCode=PW,SS,VE
  Resistor1 : fl_lib/Electrical/Electrical Elements/Resistor  R=Delta_G Ohm  i_specify=off  i_priority=None  i=0 A  i_nominal_specify=off  i_nominal_unit=A  i_nominal_value=1  v_specify=off  v_priority=None  v=0 V  v_nominal_specify=off  v_nominal_unit=V  v_nominal_value=1
      settings: SourceProductBaseCode=PW,SS,VE
  L_in : PMIOPort  Side=Left
  N_in : PMIOPort  Port=2  Side=Left
  L_out : PMIOPort  Port=3  Side=Right
  N_out : PMIOPort  Port=4  Side=Right
  connections:
  Capacitor/LConn1 -- Resistor1/LConn1 -- Inductor/RConn1 -- L_out/RConn1
  Inductor/LConn1 -- Resistor/RConn1
  L_in/RConn1 -- Resistor/LConn1
  Resistor1/RConn1 -- N_in/RConn1 -- N_out/RConn1 -- Capacitor/RConn1

== system Wanderwellen_Leitungsmodell/10 Leitungs-ESBs Nr. 1/Leitungs-ESB 2 ==
  Capacitor : fl_lib/Electrical/Electrical Elements/Capacitor  c=Delta_C F  r=1e-6 Ohm  g=0 1/Ohm  i_specify=off  i_priority=None  i=0 A  i_nominal_specify=off  i_nominal_unit=A  i_nominal_value=1  v_specify=off  v_priority=None  v=0 V  v_nominal_specify=off  v_nominal_unit=V  v_nominal_value=1  vc_specify=off  vc_priority=High  vc=0 V  vc_nominal_specify=off  vc_nominal_unit=V  vc_nominal_value=1
      settings: SourceProductBaseCode=PW,SS,VE
  Inductor : fl_lib/Electrical/Electrical Elements/Inductor  l=Delta_L H  r=0 Ohm  g=1e-9 1/Ohm  i_specify=off  i_priority=None  i=0 A  i_nominal_specify=off  i_nominal_unit=A  i_nominal_value=1  v_specify=off  v_priority=None  v=0 V  v_nominal_specify=off  v_nominal_unit=V  v_nominal_value=1  i_L_specify=off  i_L_priority=High  i_L=0 A  i_L_nominal_specify=off  i_L_nominal_unit=A  i_L_nominal_value=1
      settings: SourceProductBaseCode=PW,SS,VE
  Resistor : fl_lib/Electrical/Electrical Elements/Resistor  R=Delta_R Ohm  i_specify=off  i_priority=None  i=0 A  i_nominal_specify=off  i_nominal_unit=A  i_nominal_value=1  v_specify=off  v_priority=None  v=0 V  v_nominal_specify=off  v_nominal_unit=V  v_nominal_value=1
      settings: SourceProductBaseCode=PW,SS,VE
  Resistor1 : fl_lib/Electrical/Electrical Elements/Resistor  R=Delta_G Ohm  i_specify=off  i_priority=None  i=0 A  i_nominal_specify=off  i_nominal_unit=A  i_nominal_value=1  v_specify=off  v_priority=None  v=0 V  v_nominal_specify=off  v_nominal_unit=V  v_nominal_value=1
      settings: SourceProductBaseCode=PW,SS,VE
  L_in : PMIOPort  Side=Left
  N_in : PMIOPort  Port=2  Side=Left
  L_out : PMIOPort  Port=3  Side=Right
  N_out : PMIOPort  Port=4  Side=Right
  connections:
  Capacitor/LConn1 -- Resistor1/LConn1 -- Inductor/RConn1 -- L_out/RConn1
  Inductor/LConn1 -- Resistor/RConn1
  L_in/RConn1 -- Resistor/LConn1
  Resistor1/RConn1 -- N_in/RConn1 -- N_out/RConn1 -- Capacitor/RConn1

== system Wanderwellen_Leitungsmodell/10 Leitungs-ESBs Nr. 1/Leitungs-ESB 3 ==
  Capacitor : fl_lib/Electrical/Electrical Elements/Capacitor  c=Delta_C F  r=1e-6 Ohm  g=0 1/Ohm  i_specify=off  i_priority=None  i=0 A  i_nominal_specify=off  i_nominal_unit=A  i_nominal_value=1  v_specify=off  v_priority=None  v=0 V  v_nominal_specify=off  v_nominal_unit=V  v_nominal_value=1  vc_specify=off  vc_priority=High  vc=0 V  vc_nominal_specify=off  vc_nominal_unit=V  vc_nominal_value=1
      settings: SourceProductBaseCode=PW,SS,VE
  Inductor : fl_lib/Electrical/Electrical Elements/Inductor  l=Delta_L H  r=0 Ohm  g=1e-9 1/Ohm  i_specify=off  i_priority=None  i=0 A  i_nominal_specify=off  i_nominal_unit=A  i_nominal_value=1  v_specify=off  v_priority=None  v=0 V  v_nominal_specify=off  v_nominal_unit=V  v_nominal_value=1  i_L_specify=off  i_L_priority=High  i_L=0 A  i_L_nominal_specify=off  i_L_nominal_unit=A  i_L_nominal_value=1
      settings: SourceProductBaseCode=PW,SS,VE
  Resistor : fl_lib/Electrical/Electrical Elements/Resistor  R=Delta_R Ohm  i_specify=off  i_priority=None  i=0 A  i_nominal_specify=off  i_nominal_unit=A  i_nominal_value=1  v_specify=off  v_priority=None  v=0 V  v_nominal_specify=off  v_nominal_unit=V  v_nominal_value=1
      settings: SourceProductBaseCode=PW,SS,VE
  Resistor1 : fl_lib/Electrical/Electrical Elements/Resistor  R=Delta_G Ohm  i_specify=off  i_priority=None  i=0 A  i_nominal_specify=off  i_nominal_unit=A  i_nominal_value=1  v_specify=off  v_priority=None  v=0 V  v_nominal_specify=off  v_nominal_unit=V  v_nominal_value=1
      settings: SourceProductBaseCode=PW,SS,VE
  L_in : PMIOPort  Side=Left
  N_in : PMIOPort  Port=2  Side=Left
  L_out : PMIOPort  Port=3  Side=Right
  N_out : PMIOPort  Port=4  Side=Right
  connections:
  Capacitor/LConn1 -- Resistor1/LConn1 -- Inductor/RConn1 -- L_out/RConn1
  Inductor/LConn1 -- Resistor/RConn1
  L_in/RConn1 -- Resistor/LConn1
  Resistor1/RConn1 -- N_in/RConn1 -- N_out/RConn1 -- Capacitor/RConn1

== system Wanderwellen_Leitungsmodell/10 Leitungs-ESBs Nr. 1/Leitungs-ESB 4 ==
  Capacitor : fl_lib/Electrical/Electrical Elements/Capacitor  c=Delta_C F  r=1e-6 Ohm  g=0 1/Ohm  i_specify=off  i_priority=None  i=0 A  i_nominal_specify=off  i_nominal_unit=A  i_nominal_value=1  v_specify=off  v_priority=None  v=0 V  v_nominal_specify=off  v_nominal_unit=V  v_nominal_value=1  vc_specify=off  vc_priority=High  vc=0 V  vc_nominal_specify=off  vc_nominal_unit=V  vc_nominal_value=1
      settings: SourceProductBaseCode=PW,SS,VE
  Inductor : fl_lib/Electrical/Electrical Elements/Inductor  l=Delta_L H  r=0 Ohm  g=1e-9 1/Ohm  i_specify=off  i_priority=None  i=0 A  i_nominal_specify=off  i_nominal_unit=A  i_nominal_value=1  v_specify=off  v_priority=None  v=0 V  v_nominal_specify=off  v_nominal_unit=V  v_nominal_value=1  i_L_specify=off  i_L_priority=High  i_L=0 A  i_L_nominal_specify=off  i_L_nominal_unit=A  i_L_nominal_value=1
      settings: SourceProductBaseCode=PW,SS,VE
  Resistor : fl_lib/Electrical/Electrical Elements/Resistor  R=Delta_R Ohm  i_specify=off  i_priority=None  i=0 A  i_nominal_specify=off  i_nominal_unit=A  i_nominal_value=1  v_specify=off  v_priority=None  v=0 V  v_nominal_specify=off  v_nominal_unit=V  v_nominal_value=1
      settings: SourceProductBaseCode=PW,SS,VE
  Resistor1 : fl_lib/Electrical/Electrical Elements/Resistor  R=Delta_G Ohm  i_specify=off  i_priority=None  i=0 A  i_nominal_specify=off  i_nominal_unit=A  i_nominal_value=1  v_specify=off  v_priority=None  v=0 V  v_nominal_specify=off  v_nominal_unit=V  v_nominal_value=1
      settings: SourceProductBaseCode=PW,SS,VE
  L_in : PMIOPort  Side=Left
  N_in : PMIOPort  Port=2  Side=Left
  L_out : PMIOPort  Port=3  Side=Right
  N_out : PMIOPort  Port=4  Side=Right
  connections:
  Capacitor/LConn1 -- Resistor1/LConn1 -- Inductor/RConn1 -- L_out/RConn1
  Inductor/LConn1 -- Resistor/RConn1
  L_in/RConn1 -- Resistor/LConn1
  Resistor1/RConn1 -- N_in/RConn1 -- N_out/RConn1 -- Capacitor/RConn1

== system Wanderwellen_Leitungsmodell/10 Leitungs-ESBs Nr. 1/Leitungs-ESB 5 ==
  Capacitor : fl_lib/Electrical/Electrical Elements/Capacitor  c=Delta_C F  r=1e-6 Ohm  g=0 1/Ohm  i_specify=off  i_priority=None  i=0 A  i_nominal_specify=off  i_nominal_unit=A  i_nominal_value=1  v_specify=off  v_priority=None  v=0 V  v_nominal_specify=off  v_nominal_unit=V  v_nominal_value=1  vc_specify=off  vc_priority=High  vc=0 V  vc_nominal_specify=off  vc_nominal_unit=V  vc_nominal_value=1
      settings: SourceProductBaseCode=PW,SS,VE
  Inductor : fl_lib/Electrical/Electrical Elements/Inductor  l=Delta_L H  r=0 Ohm  g=1e-9 1/Ohm  i_specify=off  i_priority=None  i=0 A  i_nominal_specify=off  i_nominal_unit=A  i_nominal_value=1  v_specify=off  v_priority=None  v=0 V  v_nominal_specify=off  v_nominal_unit=V  v_nominal_value=1  i_L_specify=off  i_L_priority=High  i_L=0 A  i_L_nominal_specify=off  i_L_nominal_unit=A  i_L_nominal_value=1
      settings: SourceProductBaseCode=PW,SS,VE
  Resistor : fl_lib/Electrical/Electrical Elements/Resistor  R=Delta_R Ohm  i_specify=off  i_priority=None  i=0 A  i_nominal_specify=off  i_nominal_unit=A  i_nominal_value=1  v_specify=off  v_priority=None  v=0 V  v_nominal_specify=off  v_nominal_unit=V  v_nominal_value=1
      settings: SourceProductBaseCode=PW,SS,VE
  Resistor1 : fl_lib/Electrical/Electrical Elements/Resistor  R=Delta_G Ohm  i_specify=off  i_priority=None  i=0 A  i_nominal_specify=off  i_nominal_unit=A  i_nominal_value=1  v_specify=off  v_priority=None  v=0 V  v_nominal_specify=off  v_nominal_unit=V  v_nominal_value=1
      settings: SourceProductBaseCode=PW,SS,VE
  L_in : PMIOPort  Side=Left
  N_in : PMIOPort  Port=2  Side=Left
  L_out : PMIOPort  Port=3  Side=Right
  N_out : PMIOPort  Port=4  Side=Right
  connections:
  Capacitor/LConn1 -- Resistor1/LConn1 -- Inductor/RConn1 -- L_out/RConn1
  Inductor/LConn1 -- Resistor/RConn1
  L_in/RConn1 -- Resistor/LConn1
  Resistor1/RConn1 -- N_in/RConn1 -- N_out/RConn1 -- Capacitor/RConn1

== system Wanderwellen_Leitungsmodell/10 Leitungs-ESBs Nr. 1/Leitungs-ESB 6 ==
  Capacitor : fl_lib/Electrical/Electrical Elements/Capacitor  c=Delta_C F  r=1e-6 Ohm  g=0 1/Ohm  i_specify=off  i_priority=None  i=0 A  i_nominal_specify=off  i_nominal_unit=A  i_nominal_value=1  v_specify=off  v_priority=None  v=0 V  v_nominal_specify=off  v_nominal_unit=V  v_nominal_value=1  vc_specify=off  vc_priority=High  vc=0 V  vc_nominal_specify=off  vc_nominal_unit=V  vc_nominal_value=1
      settings: SourceProductBaseCode=PW,SS,VE
  Inductor : fl_lib/Electrical/Electrical Elements/Inductor  l=Delta_L H  r=0 Ohm  g=1e-9 1/Ohm  i_specify=off  i_priority=None  i=0 A  i_nominal_specify=off  i_nominal_unit=A  i_nominal_value=1  v_specify=off  v_priority=None  v=0 V  v_nominal_specify=off  v_nominal_unit=V  v_nominal_value=1  i_L_specify=off  i_L_priority=High  i_L=0 A  i_L_nominal_specify=off  i_L_nominal_unit=A  i_L_nominal_value=1
      settings: SourceProductBaseCode=PW,SS,VE
  Resistor : fl_lib/Electrical/Electrical Elements/Resistor  R=Delta_R Ohm  i_specify=off  i_priority=None  i=0 A  i_nominal_specify=off  i_nominal_unit=A  i_nominal_value=1  v_specify=off  v_priority=None  v=0 V  v_nominal_specify=off  v_nominal_unit=V  v_nominal_value=1
      settings: SourceProductBaseCode=PW,SS,VE
  Resistor1 : fl_lib/Electrical/Electrical Elements/Resistor  R=Delta_G Ohm  i_specify=off  i_priority=None  i=0 A  i_nominal_specify=off  i_nominal_unit=A  i_nominal_value=1  v_specify=off  v_priority=None  v=0 V  v_nominal_specify=off  v_nominal_unit=V  v_nominal_value=1
      settings: SourceProductBaseCode=PW,SS,VE
  L_in : PMIOPort  Side=Left
  N_in : PMIOPort  Port=2  Side=Left
  L_out : PMIOPort  Port=3  Side=Right
  N_out : PMIOPort  Port=4  Side=Right
  connections:
  Capacitor/LConn1 -- Resistor1/LConn1 -- Inductor/RConn1 -- L_out/RConn1
  Inductor/LConn1 -- Resistor/RConn1
  L_in/RConn1 -- Resistor/LConn1
  Resistor1/RConn1 -- N_in/RConn1 -- N_out/RConn1 -- Capacitor/RConn1

== system Wanderwellen_Leitungsmodell/10 Leitungs-ESBs Nr. 1/Leitungs-ESB 7 ==
  Capacitor : fl_lib/Electrical/Electrical Elements/Capacitor  c=Delta_C F  r=1e-6 Ohm  g=0 1/Ohm  i_specify=off  i_priority=None  i=0 A  i_nominal_specify=off  i_nominal_unit=A  i_nominal_value=1  v_specify=off  v_priority=None  v=0 V  v_nominal_specify=off  v_nominal_unit=V  v_nominal_value=1  vc_specify=off  vc_priority=High  vc=0 V  vc_nominal_specify=off  vc_nominal_unit=V  vc_nominal_value=1
      settings: SourceProductBaseCode=PW,SS,VE
  Inductor : fl_lib/Electrical/Electrical Elements/Inductor  l=Delta_L H  r=0 Ohm  g=1e-9 1/Ohm  i_specify=off  i_priority=None  i=0 A  i_nominal_specify=off  i_nominal_unit=A  i_nominal_value=1  v_specify=off  v_priority=None  v=0 V  v_nominal_specify=off  v_nominal_unit=V  v_nominal_value=1  i_L_specify=off  i_L_priority=High  i_L=0 A  i_L_nominal_specify=off  i_L_nominal_unit=A  i_L_nominal_value=1
      settings: SourceProductBaseCode=PW,SS,VE
  Resistor : fl_lib/Electrical/Electrical Elements/Resistor  R=Delta_R Ohm  i_specify=off  i_priority=None  i=0 A  i_nominal_specify=off  i_nominal_unit=A  i_nominal_value=1  v_specify=off  v_priority=None  v=0 V  v_nominal_specify=off  v_nominal_unit=V  v_nominal_value=1
      settings: SourceProductBaseCode=PW,SS,VE
  Resistor1 : fl_lib/Electrical/Electrical Elements/Resistor  R=Delta_G Ohm  i_specify=off  i_priority=None  i=0 A  i_nominal_specify=off  i_nominal_unit=A  i_nominal_value=1  v_specify=off  v_priority=None  v=0 V  v_nominal_specify=off  v_nominal_unit=V  v_nominal_value=1
      settings: SourceProductBaseCode=PW,SS,VE
  L_in : PMIOPort  Side=Left
  N_in : PMIOPort  Port=2  Side=Left
  L_out : PMIOPort  Port=3  Side=Right
  N_out : PMIOPort  Port=4  Side=Right
  connections:
  Capacitor/LConn1 -- Resistor1/LConn1 -- Inductor/RConn1 -- L_out/RConn1
  Inductor/LConn1 -- Resistor/RConn1
  L_in/RConn1 -- Resistor/LConn1
  Resistor1/RConn1 -- N_in/RConn1 -- N_out/RConn1 -- Capacitor/RConn1

== system Wanderwellen_Leitungsmodell/10 Leitungs-ESBs Nr. 1/Leitungs-ESB 8 ==
  Capacitor : fl_lib/Electrical/Electrical Elements/Capacitor  c=Delta_C F  r=1e-6 Ohm  g=0 1/Ohm  i_specify=off  i_priority=None  i=0 A  i_nominal_specify=off  i_nominal_unit=A  i_nominal_value=1  v_specify=off  v_priority=None  v=0 V  v_nominal_specify=off  v_nominal_unit=V  v_nominal_value=1  vc_specify=off  vc_priority=High  vc=0 V  vc_nominal_specify=off  vc_nominal_unit=V  vc_nominal_value=1
      settings: SourceProductBaseCode=PW,SS,VE
  Inductor : fl_lib/Electrical/Electrical Elements/Inductor  l=Delta_L H  r=0 Ohm  g=1e-9 1/Ohm  i_specify=off  i_priority=None  i=0 A  i_nominal_specify=off  i_nominal_unit=A  i_nominal_value=1  v_specify=off  v_priority=None  v=0 V  v_nominal_specify=off  v_nominal_unit=V  v_nominal_value=1  i_L_specify=off  i_L_priority=High  i_L=0 A  i_L_nominal_specify=off  i_L_nominal_unit=A  i_L_nominal_value=1
      settings: SourceProductBaseCode=PW,SS,VE
  Resistor : fl_lib/Electrical/Electrical Elements/Resistor  R=Delta_R Ohm  i_specify=off  i_priority=None  i=0 A  i_nominal_specify=off  i_nominal_unit=A  i_nominal_value=1  v_specify=off  v_priority=None  v=0 V  v_nominal_specify=off  v_nominal_unit=V  v_nominal_value=1
      settings: SourceProductBaseCode=PW,SS,VE
  Resistor1 : fl_lib/Electrical/Electrical Elements/Resistor  R=Delta_G Ohm  i_specify=off  i_priority=None  i=0 A  i_nominal_specify=off  i_nominal_unit=A  i_nominal_value=1  v_specify=off  v_priority=None  v=0 V  v_nominal_specify=off  v_nominal_unit=V  v_nominal_value=1
      settings: SourceProductBaseCode=PW,SS,VE
  L_in : PMIOPort  Side=Left
  N_in : PMIOPort  Port=2  Side=Left
  L_out : PMIOPort  Port=3  Side=Right
  N_out : PMIOPort  Port=4  Side=Right
  connections:
  Capacitor/LConn1 -- Resistor1/LConn1 -- Inductor/RConn1 -- L_out/RConn1
  Inductor/LConn1 -- Resistor/RConn1
  L_in/RConn1 -- Resistor/LConn1
  Resistor1/RConn1 -- N_in/RConn1 -- N_out/RConn1 -- Capacitor/RConn1

== system Wanderwellen_Leitungsmodell/10 Leitungs-ESBs Nr. 1/Leitungs-ESB 9 ==
  Capacitor : fl_lib/Electrical/Electrical Elements/Capacitor  c=Delta_C F  r=1e-6 Ohm  g=0 1/Ohm  i_specify=off  i_priority=None  i=0 A  i_nominal_specify=off  i_nominal_unit=A  i_nominal_value=1  v_specify=off  v_priority=None  v=0 V  v_nominal_specify=off  v_nominal_unit=V  v_nominal_value=1  vc_specify=off  vc_priority=High  vc=0 V  vc_nominal_specify=off  vc_nominal_unit=V  vc_nominal_value=1
      settings: SourceProductBaseCode=PW,SS,VE
  Inductor : fl_lib/Electrical/Electrical Elements/Inductor  l=Delta_L H  r=0 Ohm  g=1e-9 1/Ohm  i_specify=off  i_priority=None  i=0 A  i_nominal_specify=off  i_nominal_unit=A  i_nominal_value=1  v_specify=off  v_priority=None  v=0 V  v_nominal_specify=off  v_nominal_unit=V  v_nominal_value=1  i_L_specify=off  i_L_priority=High  i_L=0 A  i_L_nominal_specify=off  i_L_nominal_unit=A  i_L_nominal_value=1
      settings: SourceProductBaseCode=PW,SS,VE
  Resistor : fl_lib/Electrical/Electrical Elements/Resistor  R=Delta_R Ohm  i_specify=off  i_priority=None  i=0 A  i_nominal_specify=off  i_nominal_unit=A  i_nominal_value=1  v_specify=off  v_priority=None  v=0 V  v_nominal_specify=off  v_nominal_unit=V  v_nominal_value=1
      settings: SourceProductBaseCode=PW,SS,VE
  Resistor1 : fl_lib/Electrical/Electrical Elements/Resistor  R=Delta_G Ohm  i_specify=off  i_priority=None  i=0 A  i_nominal_specify=off  i_nominal_unit=A  i_nominal_value=1  v_specify=off  v_priority=None  v=0 V  v_nominal_specify=off  v_nominal_unit=V  v_nominal_value=1
      settings: SourceProductBaseCode=PW,SS,VE
  L_in : PMIOPort  Side=Left
  N_in : PMIOPort  Port=2  Side=Left
  L_out : PMIOPort  Port=3  Side=Right
  N_out : PMIOPort  Port=4  Side=Right
  connections:
  Capacitor/LConn1 -- Resistor1/LConn1 -- Inductor/RConn1 -- L_out/RConn1
  Inductor/LConn1 -- Resistor/RConn1
  L_in/RConn1 -- Resistor/LConn1
  Resistor1/RConn1 -- N_in/RConn1 -- N_out/RConn1 -- Capacitor/RConn1

== system Wanderwellen_Leitungsmodell/10 Leitungs-ESBs Nr. 10/Leitungs-ESB 1 ==
  Capacitor : fl_lib/Electrical/Electrical Elements/Capacitor  c=Delta_C F  r=1e-6 Ohm  g=0 1/Ohm  i_specify=off  i_priority=None  i=0 A  i_nominal_specify=off  i_nominal_unit=A  i_nominal_value=1  v_specify=off  v_priority=None  v=0 V  v_nominal_specify=off  v_nominal_unit=V  v_nominal_value=1  vc_specify=off  vc_priority=High  vc=0 V  vc_nominal_specify=off  vc_nominal_unit=V  vc_nominal_value=1
      settings: SourceProductBaseCode=PW,SS,VE
  Inductor : fl_lib/Electrical/Electrical Elements/Inductor  l=Delta_L H  r=0 Ohm  g=1e-9 1/Ohm  i_specify=off  i_priority=None  i=0 A  i_nominal_specify=off  i_nominal_unit=A  i_nominal_value=1  v_specify=off  v_priority=None  v=0 V  v_nominal_specify=off  v_nominal_unit=V  v_nominal_value=1  i_L_specify=off  i_L_priority=High  i_L=0 A  i_L_nominal_specify=off  i_L_nominal_unit=A  i_L_nominal_value=1
      settings: SourceProductBaseCode=PW,SS,VE
  Resistor : fl_lib/Electrical/Electrical Elements/Resistor  R=Delta_R Ohm  i_specify=off  i_priority=None  i=0 A  i_nominal_specify=off  i_nominal_unit=A  i_nominal_value=1  v_specify=off  v_priority=None  v=0 V  v_nominal_specify=off  v_nominal_unit=V  v_nominal_value=1
      settings: SourceProductBaseCode=PW,SS,VE
  Resistor1 : fl_lib/Electrical/Electrical Elements/Resistor  R=Delta_G Ohm  i_specify=off  i_priority=None  i=0 A  i_nominal_specify=off  i_nominal_unit=A  i_nominal_value=1  v_specify=off  v_priority=None  v=0 V  v_nominal_specify=off  v_nominal_unit=V  v_nominal_value=1
      settings: SourceProductBaseCode=PW,SS,VE
  L_in : PMIOPort  Side=Left
  N_in : PMIOPort  Port=2  Side=Left
  L_out : PMIOPort  Port=3  Side=Right
  N_out : PMIOPort  Port=4  Side=Right
  connections:
  Capacitor/LConn1 -- Resistor1/LConn1 -- Inductor/RConn1 -- L_out/RConn1
  Inductor/LConn1 -- Resistor/RConn1
  L_in/RConn1 -- Resistor/LConn1
  Resistor1/RConn1 -- N_in/RConn1 -- N_out/RConn1 -- Capacitor/RConn1

== system Wanderwellen_Leitungsmodell/10 Leitungs-ESBs Nr. 10/Leitungs-ESB 10 ==
  Capacitor : fl_lib/Electrical/Electrical Elements/Capacitor  c=Delta_C F  r=1e-6 Ohm  g=0 1/Ohm  i_specify=off  i_priority=None  i=0 A  i_nominal_specify=off  i_nominal_unit=A  i_nominal_value=1  v_specify=off  v_priority=None  v=0 V  v_nominal_specify=off  v_nominal_unit=V  v_nominal_value=1  vc_specify=off  vc_priority=High  vc=0 V  vc_nominal_specify=off  vc_nominal_unit=V  vc_nominal_value=1
      settings: SourceProductBaseCode=PW,SS,VE
  Inductor : fl_lib/Electrical/Electrical Elements/Inductor  l=Delta_L H  r=0 Ohm  g=1e-9 1/Ohm  i_specify=off  i_priority=None  i=0 A  i_nominal_specify=off  i_nominal_unit=A  i_nominal_value=1  v_specify=off  v_priority=None  v=0 V  v_nominal_specify=off  v_nominal_unit=V  v_nominal_value=1  i_L_specify=off  i_L_priority=High  i_L=0 A  i_L_nominal_specify=off  i_L_nominal_unit=A  i_L_nominal_value=1
      settings: SourceProductBaseCode=PW,SS,VE
  Resistor : fl_lib/Electrical/Electrical Elements/Resistor  R=Delta_R Ohm  i_specify=off  i_priority=None  i=0 A  i_nominal_specify=off  i_nominal_unit=A  i_nominal_value=1  v_specify=off  v_priority=None  v=0 V  v_nominal_specify=off  v_nominal_unit=V  v_nominal_value=1
      settings: SourceProductBaseCode=PW,SS,VE
  Resistor1 : fl_lib/Electrical/Electrical Elements/Resistor  R=Delta_G Ohm  i_specify=off  i_priority=None  i=0 A  i_nominal_specify=off  i_nominal_unit=A  i_nominal_value=1  v_specify=off  v_priority=None  v=0 V  v_nominal_specify=off  v_nominal_unit=V  v_nominal_value=1
      settings: SourceProductBaseCode=PW,SS,VE
  L_in : PMIOPort  Side=Left
  N_in : PMIOPort  Port=2  Side=Left
  L_out : PMIOPort  Port=3  Side=Right
  N_out : PMIOPort  Port=4  Side=Right
  connections:
  Capacitor/LConn1 -- Resistor1/LConn1 -- Inductor/RConn1 -- L_out/RConn1
  Inductor/LConn1 -- Resistor/RConn1
  L_in/RConn1 -- Resistor/LConn1
  Resistor1/RConn1 -- N_in/RConn1 -- N_out/RConn1 -- Capacitor/RConn1
